simulink model "SWC1"  (R2022b)
settings: Solver=FixedStepAuto  StartTime=0.0  StopTime=10.0  RelTol=1e-3  EnableMultiTasking=on
settings Model: Creator=EDKI  LastModifiedBy=EDKI

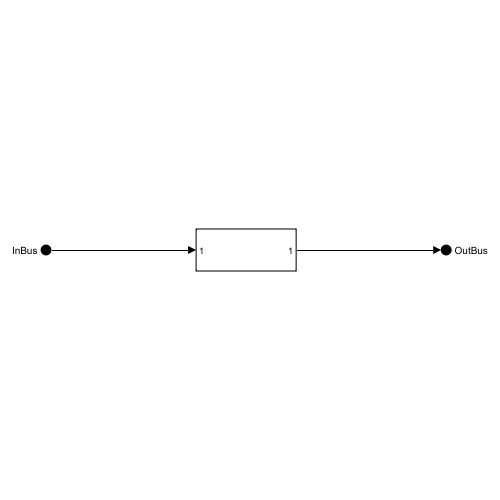
[thumbnail: Simulink's stored preview of the top-level diagram]
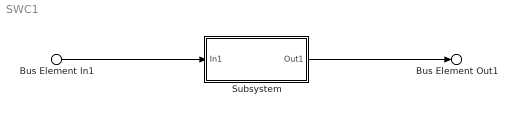
== system SWC1 ==
  Bus Element In1 : Inport  PortName=InBus
  Subsystem : Subsystem
  Bus Element Out1 : Outport  PortName=OutBus
  wires:
  Bus Element In1/1 -> Subsystem/1(In1)
  Subsystem/1(Out1) -> Bus Element Out1/1

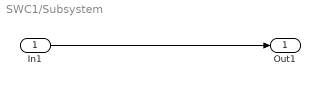
== system SWC1/Subsystem ==
  In1 : Inport
  Out1 : Outport
  wires:
  In1/1 -> Out1/1
